simulink model "AttitudeControl_tune"  (R2017b)
settings: Solver=ode4  StartTime=0.0  StopTime=10  FixedStep=0.001  RelTol=1e-3
InitFcn:
  | Init_control
undefined symbols (not defined in the file): DiscIntNeverNeededParam, Kd_PITCH_AngleRate, Kd_ROLL_AngleRate, Kd_YAW_AngleRate, Ki_PITCH_AngleRate, Ki_ROLL_AngleRate, Ki_YAW_AngleRate, Kp_PITCH_ANGLE, Kp_PITCH_AngleRate, Kp_ROLL_ANGLE, Kp_ROLL_AngleRate, Kp_YAW_AngleRate, MAX_CONTROL_ANGLE_RATE_PITCH, MAX_CONTROL_ANGLE_RATE_ROLL, ModelInit_AngEuler, ModelInit_PosE, ModelInit_Rads, ModelInit_RateB, ModelInit_VelB, ModelParam_envGravityAcc, ModelParam_motorCr, ModelParam_motorJm, ModelParam_motorT, ModelParam_motorWb, ModelParam_rotorCm, ModelParam_rotorCt, ModelParam_uavCCm, ModelParam_uavCd, ModelParam_uavJ, ModelParam_uavMass, ModelParam_uavR, Saturation_I_RP_Max, Saturation_I_RP_Min, Saturation_I_Y_Max, Saturation_I_Y_Min
libraries: simulink x3, sharedutil x2
settings Model: Creator=wsh  LastModifiedBy=Mr Wang
settings OptimizationCC: MaxStackSize=64
settings DebuggingCC: ParameterTunabilityLossMsg=error
settings HardwareCC: ProdBitPerPointer=32  ProdBitPerSizeT=32  ProdBitPerPtrDiffT=32  ProdLargestAtomicInteger=Long  ProdLargestAtomicFloat=Double  ProdWordSize=32  ProdHWDeviceType=ARM Compatible->ARM Cortex
settings SFSimCC: MATLABDynamicMemAlloc=off
settings RTWCC: SystemTargetFile=ert.tlc  HardwareBoard=Pixhawk PX4  TemplateMakefile=ert_default_tmf  GenerateReport=on  Toolchain=Pixhawk Toolchain  IncludeHyperlinkInReport=on  LaunchReport=on  GenerateTraceInfo=on  GenerateTraceReport=on  GenerateTraceReportSl=on  GenerateTraceReportSf=on  GenerateTraceReportEml=on
settings CodeAppCC: ForceParamTrailComments=on  IgnoreCustomStorageClasses=off  OperatorAnnotations=on  SimulinkDataObjDesc=on  SFDataObjDesc=on  MATLABFcnDesc=on  InsertBlockDesc=on  StateflowObjectComments=on  MATLABSourceComments=on
settings ERTTargetCC: MultiwordLength=2048  ERTCustomFileTemplate=PX4_codertarget_file_process.tlc

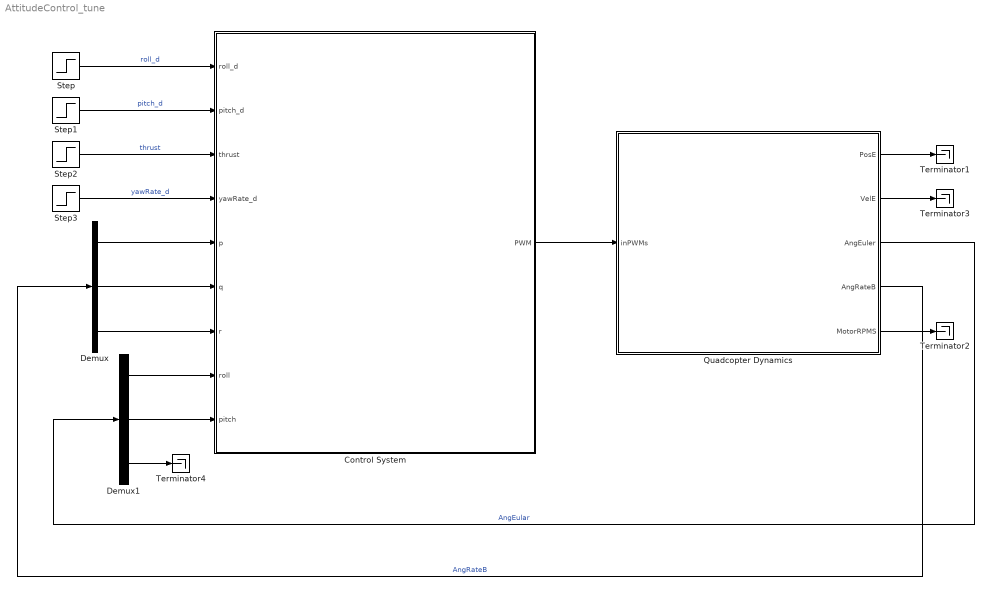
== system AttitudeControl_tune ==
  Control System : Subsystem
      mask Display: image('icon\pixhawk.png');
  Demux : Demux  Outputs=3
  Demux1 : Demux  Outputs=3
  Quadcopter Dynamics : Subsystem
      mask Display: image('./icon/F450.png');
  Step : Step  Time=0  After=0  SampleTime=0
  Step1 : Step  Time=0  After=0  SampleTime=0
  Step2 : Step  Time=0  After=0.6085  SampleTime=0
  Step3 : Step  Time=0  After=0  SampleTime=0
  Terminator{1..4} (4 alike) : Terminator
  wires:
  Quadcopter Dynamics/3(AngEuler) -> Demux1/1  "AngEular"
  Quadcopter Dynamics/4(AngRateB) -> Demux/1  "AngRateB"
  Demux/1 -> Control System/5(p)
  Demux/2 -> Control System/6(q)
  Demux/3 -> Control System/7(r)
  Demux1/1 -> Control System/8(roll)
  Demux1/3 -> Terminator4/1
  Demux1/2 -> Control System/9(pitch)
  Quadcopter Dynamics/1(PosE) -> Terminator1/1
  Quadcopter Dynamics/2(VelE) -> Terminator3/1
  Step1/1 -> Control System/2(pitch_d)  "pitch_d"
  Step/1 -> Control System/1(roll_d)  "roll_d"
  Step3/1 -> Control System/4(yawRate_d)  "yawRate_d"
  Step2/1 -> Control System/3(thrust)  "thrust"
  Quadcopter Dynamics/5(MotorRPMS) -> Terminator2/1
  Control System/1(PWM) -> Quadcopter Dynamics/1(inPWMs)

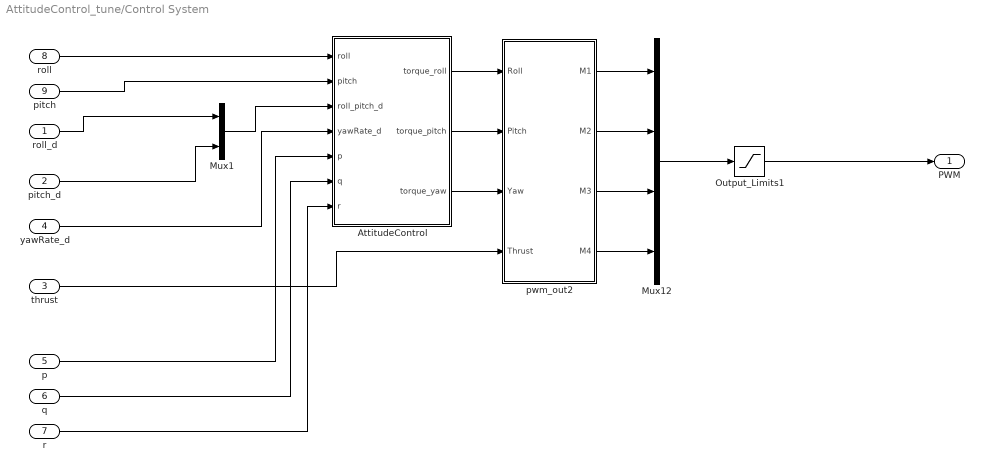
== system AttitudeControl_tune/Control System ==
  roll_d : Inport  PortDimensions=1
  pitch_d : Inport  Port=2  PortDimensions=1
  thrust : Inport  Port=3  PortDimensions=1
  yawRate_d : Inport  Port=4  PortDimensions=1
  p : Inport  Port=5  PortDimensions=1
  q : Inport  Port=6  PortDimensions=1
  r : Inport  Port=7  PortDimensions=1
  roll : Inport  Port=8  PortDimensions=1
  pitch : Inport  Port=9  PortDimensions=1
  AttitudeControl : Subsystem
  Mux1 : Mux  Inputs=2
  Mux12 : Mux
  Output_Limits1 : Saturate  UpperLimit=2000  LowerLimit=1000  LinearizeAsGain=off
  pwm_out2 : MATLAB Function  SystemSampleTime=0.004
  PWM : Outport
  wires:
  thrust/1 -> pwm_out2/4(Thrust)
  Mux12/1 -> Output_Limits1/1
  AttitudeControl/2(torque_pitch) -> pwm_out2/2(Pitch)
  AttitudeControl/1(torque_roll) -> pwm_out2/1(Roll)
  pwm_out2/1(M1) -> Mux12/1
  pwm_out2/3(M3) -> Mux12/3
  pwm_out2/2(M2) -> Mux12/2
  r/1 -> AttitudeControl/7(r)
  AttitudeControl/3(torque_yaw) -> pwm_out2/3(Yaw)
  Mux1/1 -> AttitudeControl/3(roll_pitch_d)
  q/1 -> AttitudeControl/6(q)
  yawRate_d/1 -> AttitudeControl/4(yawRate_d)
  p/1 -> AttitudeControl/5(p)
  pwm_out2/4(M4) -> Mux12/4
  pitch/1 -> AttitudeControl/2(pitch)
  roll/1 -> AttitudeControl/1(roll)
  Output_Limits1/1 -> PWM/1
  roll_d/1 -> Mux1/1
  pitch_d/1 -> Mux1/2

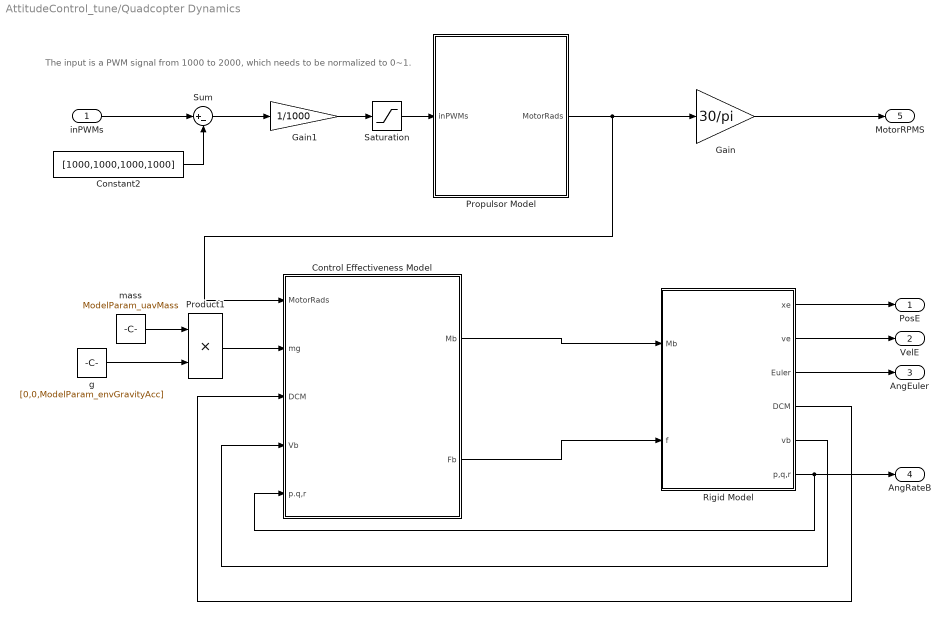
== system AttitudeControl_tune/Quadcopter Dynamics ==
  note: The input is a PWM signal from 1000 to 2000,
      | which needs to be normalized to 0~1.
  inPWMs : Inport
  Constant2 : Constant  Value=[1000,1000,1000,1000]
  Control Effectiveness Model : Subsystem
  Gain : Gain  Gain=30/pi
  Gain1 : Gain  Gain=1/1000
  Product1 : Product
  Propulsor Model : Subsystem
  Rigid Model : Subsystem
  Saturation : Saturate  UpperLimit=1  LowerLimit=0
  Sum : Sum  Inputs=|+-
  g : Constant  Value=[0,0,ModelParam_envGravityAcc]
  mass : Constant  Value=ModelParam_uavMass
  PosE : Outport
  VelE : Outport  Port=2
  AngEuler : Outport  Port=3
  AngRateB : Outport  Port=4
  MotorRPMS : Outport  Port=5
  wires:
  Saturation/1 -> Propulsor Model/1(inPWMs)
  Rigid Model/6("p,q,r ") -> Control Effectiveness Model/5(p.q,r), AngRateB/1
  mass/1 -> Product1/1
  Rigid Model/4(DCM) -> Control Effectiveness Model/3(DCM)
  Propulsor Model/1(MotorRads) -> Gain/1, Control Effectiveness Model/1(MotorRads)
  Gain1/1 -> Saturation/1
  Rigid Model/2(ve) -> VelE/1
  Sum/1 -> Gain1/1
  Product1/1 -> Control Effectiveness Model/2(mg)
  Rigid Model/5("vb ") -> Control Effectiveness Model/4(Vb)
  Rigid Model/1("xe ") -> PosE/1
  Rigid Model/3(Euler) -> AngEuler/1
  Control Effectiveness Model/1(Mb) -> Rigid Model/1(Mb)
  inPWMs/1 -> Sum/1
  Control Effectiveness Model/2(Fb) -> Rigid Model/2(f)
  Constant2/1 -> Sum/2
  g/1 -> Product1/2
  Gain/1 -> MotorRPMS/1

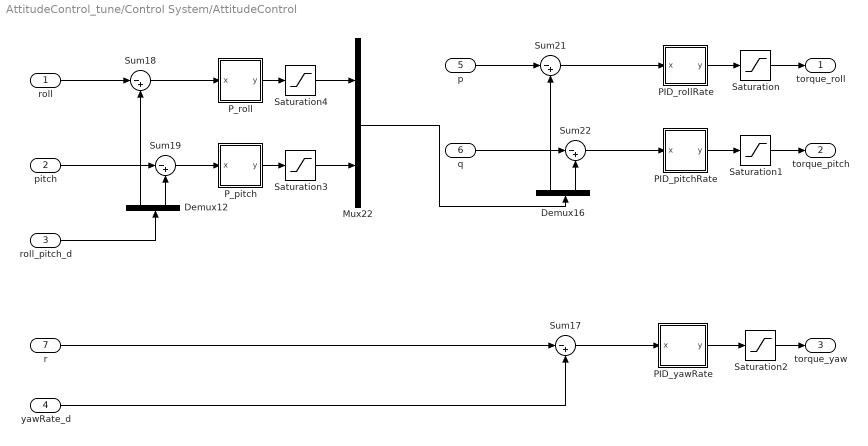
== system AttitudeControl_tune/Control System/AttitudeControl ==
  roll : Inport
  pitch : Inport  Port=2
  roll_pitch_d : Inport  Port=3
  yawRate_d : Inport  Port=4
  p : Inport  Port=5
  q : Inport  Port=6
  r : Inport  Port=7
  Demux12 : Demux  Outputs=2
  Demux16 : Demux  Outputs=2
  Mux22 : Mux  Inputs=2
  PID_pitchRate : Subsystem
  PID_rollRate : Subsystem
  PID_yawRate : Subsystem
  "P_pitch " : Subsystem
  "P_roll " : Subsystem
  Saturation : Saturate  UpperLimit=1  LowerLimit=-1
  Saturation1 : Saturate  UpperLimit=1  LowerLimit=-1
  Saturation2 : Saturate
  Saturation3 : Saturate  UpperLimit=MAX_CONTROL_ANGLE_RATE_PITCH  LowerLimit=-MAX_CONTROL_ANGLE_RATE_PITCH
  Saturation4 : Saturate  UpperLimit=MAX_CONTROL_ANGLE_RATE_ROLL  LowerLimit=-MAX_CONTROL_ANGLE_RATE_ROLL
  Sum{17..19,21..22} (5 alike) : Sum  Inputs=|-+
  torque_roll : Outport
  torque_pitch : Outport  Port=2
  torque_yaw : Outport  Port=3
  wires:
  r/1 -> Sum17/1
  Sum19/1 -> "P_pitch "/1(x)
  "P_pitch "/1(y) -> Saturation3/1
  "P_roll "/1(y) -> Saturation4/1
  roll/1 -> Sum18/1
  pitch/1 -> Sum19/1
  Sum18/1 -> "P_roll "/1(x)
  Sum22/1 -> PID_pitchRate/1(x)
  Sum17/1 -> PID_yawRate/1(x)
  p/1 -> Sum21/1
  q/1 -> Sum22/1
  Sum21/1 -> PID_rollRate/1(x)
  PID_pitchRate/1(y) -> Saturation1/1
  PID_rollRate/1(y) -> Saturation/1
  PID_yawRate/1(y) -> Saturation2/1
  roll_pitch_d/1 -> Demux12/1
  Saturation1/1 -> torque_pitch/1
  yawRate_d/1 -> Sum17/2
  Mux22/1 -> Demux16/1
  Saturation4/1 -> Mux22/1
  Saturation3/1 -> Mux22/2
  Saturation/1 -> torque_roll/1
  Saturation2/1 -> torque_yaw/1
  Demux16/1 -> Sum21/2
  Demux12/2 -> Sum19/2
  Demux12/1 -> Sum18/2
  Demux16/2 -> Sum22/2

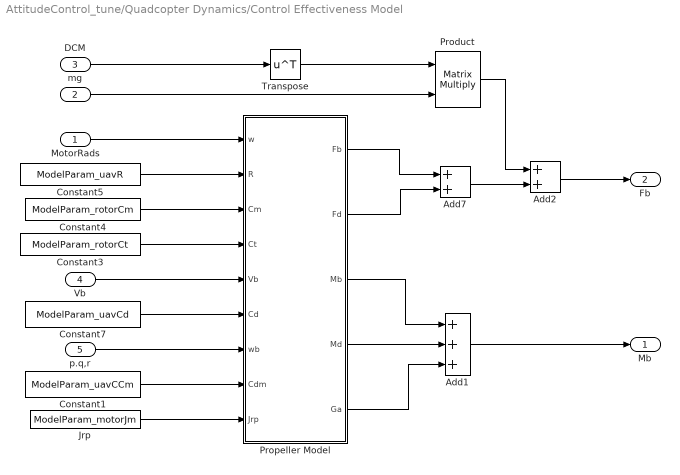
== system AttitudeControl_tune/Quadcopter Dynamics/Control Effectiveness Model ==
  MotorRads : Inport
  mg : Inport  Port=2
  DCM : Inport  Port=3
  Vb : Inport  Port=4
  p.q,r : Inport  Port=5
  Add1 : Sum  Inputs=+++
  Add2 : Sum
  Add7 : Sum
  Constant1 : Constant  Value=ModelParam_uavCCm
  Constant3 : Constant  Value=ModelParam_rotorCt
  Constant4 : Constant  Value=ModelParam_rotorCm
  Constant5 : Constant  Value=ModelParam_uavR
  Constant7 : Constant  Value=ModelParam_uavCd
  Jrp : Constant  Value=ModelParam_motorJm
  Product : Product  Multiplication=Matrix(*)
  Propeller Model : MATLAB Function  TreatAsAtomicUnit=on
  Transpose : Math  Operator=transpose  SaturateOnIntegerOverflow=on
  Mb : Outport
  Fb : Outport  Port=2
  wires:
  Add2/1 -> Fb/1
  Constant3/1 -> Propeller Model/4(Ct)
  Propeller Model/2(Fd) -> Add7/2
  Add7/1 -> Add2/2
  Propeller Model/1(Fb) -> Add7/1
  Product/1 -> Add2/1
  mg/1 -> Product/2
  DCM/1 -> Transpose/1
  Constant7/1 -> Propeller Model/6(Cd)
  Vb/1 -> Propeller Model/5(Vb)
  Constant5/1 -> Propeller Model/2(R)
  Constant4/1 -> Propeller Model/3(Cm)
  MotorRads/1 -> Propeller Model/1(w)
  Transpose/1 -> Product/1
  Propeller Model/3(Mb) -> Add1/1
  Propeller Model/4(Md) -> Add1/2
  Add1/1 -> Mb/1
  p.q,r/1 -> Propeller Model/7(wb)
  Constant1/1 -> Propeller Model/8(Cdm)
  Jrp/1 -> Propeller Model/9(Jrp)
  Propeller Model/5(Ga) -> Add1/3

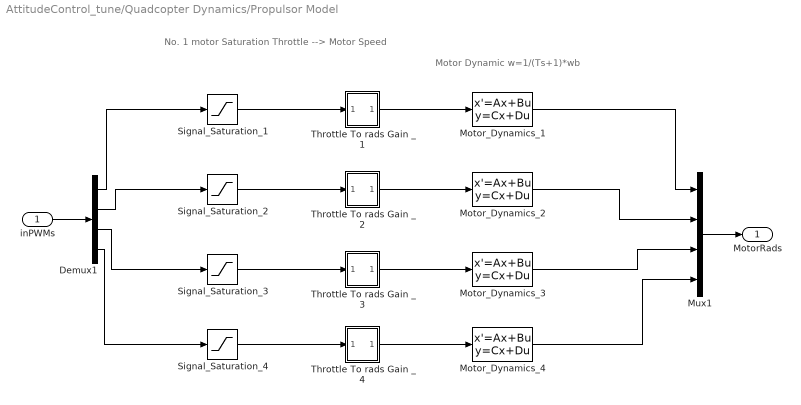
== system AttitudeControl_tune/Quadcopter Dynamics/Propulsor Model ==
  note: Motor Dynamic
      | w=1/(Ts+1)*wb
  note: No. 1 motor
      |
      |          Saturation             Throttle --> Motor Speed
  inPWMs : Inport
  Demux1 : Demux
  Motor_Dynamics_{1..4} (4 alike) : StateSpace  A=-1/ModelParam_motorT  C=1/ModelParam_motorT  D=0  InitialCondition=ModelInit_Rads*ModelParam_motorT
  Mux1 : Mux
  Signal_Saturation_{1..4} (4 alike) : Saturate  UpperLimit=1  LowerLimit=0
  Throttle To rads Gain _1 : Subsystem
  Throttle To rads Gain _2 : Subsystem
  Throttle To rads Gain _3 : Subsystem
  Throttle To rads Gain _4 : Subsystem
  MotorRads : Outport
  wires:
  Throttle To rads Gain _4/1(Out5) -> Motor_Dynamics_4/1
  Signal_Saturation_4/1 -> Throttle To rads Gain _4/1(In5)
  Signal_Saturation_3/1 -> Throttle To rads Gain _3/1(In5)
  Signal_Saturation_2/1 -> Throttle To rads Gain _2/1(In5)
  Motor_Dynamics_4/1 -> Mux1/4
  Motor_Dynamics_3/1 -> Mux1/3
  Motor_Dynamics_2/1 -> Mux1/2
  Motor_Dynamics_1/1 -> Mux1/1
  Signal_Saturation_1/1 -> Throttle To rads Gain _1/1(In5)
  Mux1/1 -> MotorRads/1
  Throttle To rads Gain _3/1(Out5) -> Motor_Dynamics_3/1
  Throttle To rads Gain _2/1(Out5) -> Motor_Dynamics_2/1
  Throttle To rads Gain _1/1(Out5) -> Motor_Dynamics_1/1
  inPWMs/1 -> Demux1/1
  Demux1/4 -> Signal_Saturation_4/1
  Demux1/3 -> Signal_Saturation_3/1
  Demux1/2 -> Signal_Saturation_2/1
  Demux1/1 -> Signal_Saturation_1/1

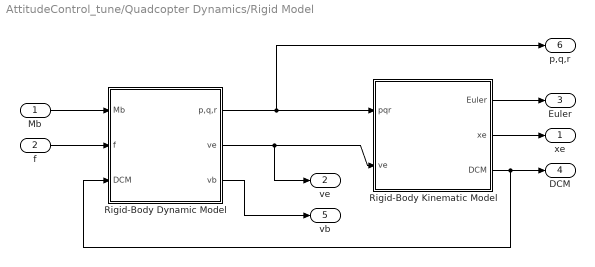
== system AttitudeControl_tune/Quadcopter Dynamics/Rigid Model ==
  Mb : Inport
  f : Inport  Port=2
  Rigid-Body Dynamic Model : Subsystem
  "Rigid-Body Kinematic Model " : Subsystem
  "xe " : Outport
  ve : Outport  Port=2
  Euler : Outport  Port=3
  DCM : Outport  Port=4
  "vb " : Outport  Port=5
  "p,q,r " : Outport  Port=6
  wires:
  Rigid-Body Dynamic Model/1("p,q,r ") -> "Rigid-Body Kinematic Model "/1(pqr), "p,q,r "/1
  "Rigid-Body Kinematic Model "/1(Euler) -> Euler/1
  "Rigid-Body Kinematic Model "/3(DCM) -> Rigid-Body Dynamic Model/3(DCM), DCM/1
  Mb/1 -> Rigid-Body Dynamic Model/1(Mb)
  f/1 -> Rigid-Body Dynamic Model/2(f)
  Rigid-Body Dynamic Model/2(ve) -> "Rigid-Body Kinematic Model "/2(ve), ve/1
  Rigid-Body Dynamic Model/3("vb ") -> "vb "/1
  "Rigid-Body Kinematic Model "/2("xe ") -> "xe "/1

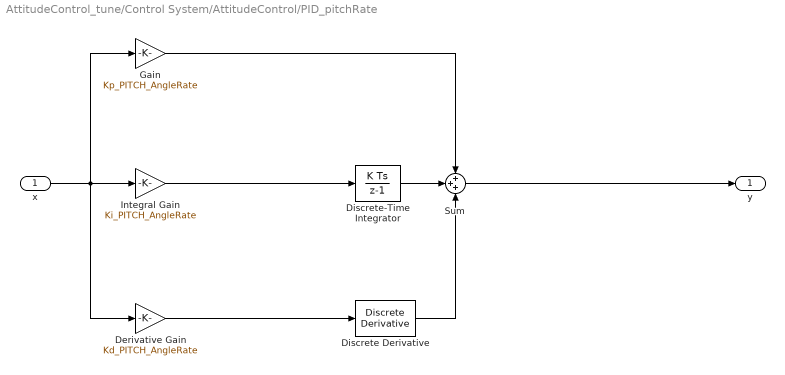
== system AttitudeControl_tune/Control System/AttitudeControl/PID_pitchRate ==
  x : Inport
  Derivative Gain : Gain  DisableCoverage=on  Gain=Kd_PITCH_AngleRate  ParamMin=-100  ParamMax=100  OutMin=-100  OutMax=100
  Discrete Derivative : simulink/Discrete/Discrete Derivative  gainval=1.0  ICPrevScaledInput=0.0  OutMin=[]  OutMax=[]  OutDataType=fixdt(1, 16)  OutScaling=2^-10  DoSatur=off
  Discrete-Time Integrator : DiscreteIntegrator  InitialConditionSetting=State (most efficient)  SampleTime=-1  LimitOutput=on  UpperSaturationLimit=Saturation_I_RP_Max  LowerSaturationLimit=Saturation_I_RP_Min  ICPrevOutput=DiscIntNeverNeededParam  ICPrevScaledInput=DiscIntNeverNeededParam
  Gain : Gain  Gain=Kp_PITCH_AngleRate
  Integral Gain : Gain  DisableCoverage=on  Gain=Ki_PITCH_AngleRate
  Sum : Sum  Inputs=+++
  y : Outport  InitialOutput=0
  wires:
  Discrete-Time Integrator/1 -> Sum/2
  Discrete Derivative/1 -> Sum/3
  Sum/1 -> y/1
  Gain/1 -> Sum/1
  Derivative Gain/1 -> Discrete Derivative/1
  Integral Gain/1 -> Discrete-Time Integrator/1
  x/1 -> Derivative Gain/1, Integral Gain/1, Gain/1

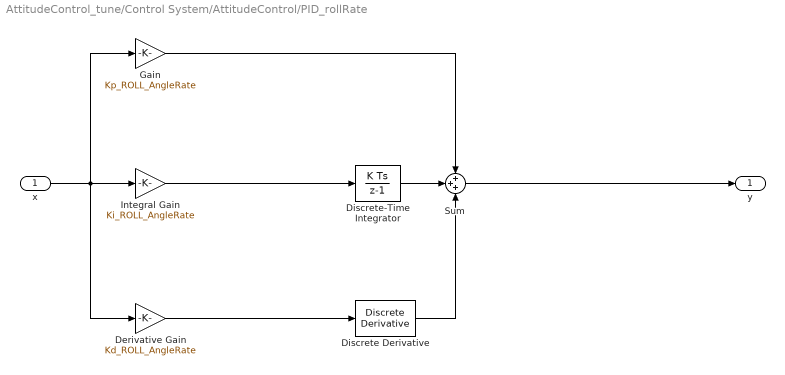
== system AttitudeControl_tune/Control System/AttitudeControl/PID_rollRate ==
  x : Inport
  Derivative Gain : Gain  DisableCoverage=on  Gain=Kd_ROLL_AngleRate  ParamMin=-100  ParamMax=100  OutMin=-100  OutMax=100
  Discrete Derivative : simulink/Discrete/Discrete Derivative  gainval=1.0  ICPrevScaledInput=0.0  OutMin=[]  OutMax=[]  OutDataType=fixdt(1, 16)  OutScaling=2^-10  DoSatur=off
  Discrete-Time Integrator : DiscreteIntegrator  InitialConditionSetting=State (most efficient)  SampleTime=-1  LimitOutput=on  UpperSaturationLimit=Saturation_I_RP_Max  LowerSaturationLimit=Saturation_I_RP_Min  ICPrevOutput=DiscIntNeverNeededParam  ICPrevScaledInput=DiscIntNeverNeededParam
  Gain : Gain  Gain=Kp_ROLL_AngleRate
  Integral Gain : Gain  DisableCoverage=on  Gain=Ki_ROLL_AngleRate
  Sum : Sum  Inputs=+++
  y : Outport  InitialOutput=0
  wires:
  x/1 -> Gain/1, Integral Gain/1, Derivative Gain/1
  Integral Gain/1 -> Discrete-Time Integrator/1
  Derivative Gain/1 -> Discrete Derivative/1
  Gain/1 -> Sum/1
  Sum/1 -> y/1
  Discrete Derivative/1 -> Sum/3
  Discrete-Time Integrator/1 -> Sum/2

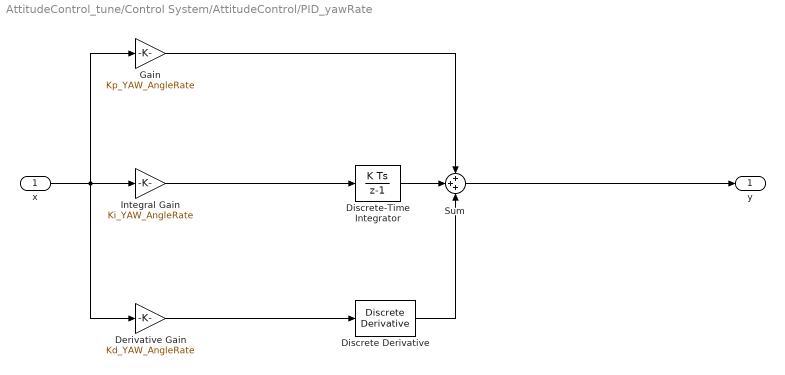
== system AttitudeControl_tune/Control System/AttitudeControl/PID_yawRate ==
  x : Inport
  Derivative Gain : Gain  DisableCoverage=on  Gain=Kd_YAW_AngleRate  ParamMin=-100  ParamMax=100  OutMin=-100  OutMax=100
  Discrete Derivative : simulink/Discrete/Discrete Derivative  gainval=1.0  ICPrevScaledInput=0.0  OutMin=[]  OutMax=[]  OutDataType=fixdt(1, 16)  OutScaling=2^-10  DoSatur=off
  Discrete-Time Integrator : DiscreteIntegrator  InitialConditionSetting=State (most efficient)  SampleTime=-1  LimitOutput=on  UpperSaturationLimit=Saturation_I_Y_Max  LowerSaturationLimit=Saturation_I_Y_Min  ICPrevOutput=DiscIntNeverNeededParam  ICPrevScaledInput=DiscIntNeverNeededParam
  Gain : Gain  Gain=Kp_YAW_AngleRate
  Integral Gain : Gain  DisableCoverage=on  Gain=Ki_YAW_AngleRate
  Sum : Sum  Inputs=+++
  y : Outport  InitialOutput=0
  wires:
  x/1 -> Gain/1, Integral Gain/1, Derivative Gain/1
  Integral Gain/1 -> Discrete-Time Integrator/1
  Derivative Gain/1 -> Discrete Derivative/1
  Gain/1 -> Sum/1
  Sum/1 -> y/1
  Discrete Derivative/1 -> Sum/3
  Discrete-Time Integrator/1 -> Sum/2

== system AttitudeControl_tune/Control System/AttitudeControl/P_pitch  ==
  x : Inport
  Gain : Gain  Gain=Kp_PITCH_ANGLE
  y : Outport  InitialOutput=0
  wires:
  x/1 -> Gain/1
  Gain/1 -> y/1

== system AttitudeControl_tune/Control System/AttitudeControl/P_roll  ==
  x : Inport
  Gain : Gain  Gain=Kp_ROLL_ANGLE
  y : Outport  InitialOutput=0
  wires:
  Gain/1 -> y/1
  x/1 -> Gain/1

== system AttitudeControl_tune/Quadcopter Dynamics/Propulsor Model/Throttle To rads Gain _1 ==
  In5 : Inport
  Constant : Constant  Value=ModelParam_motorWb
  Gain : Gain  Gain=ModelParam_motorCr
  Sum1 : Sum  Inputs=++|
  Out5 : Outport
  wires:
  Constant/1 -> Sum1/1
  Gain/1 -> Sum1/2
  In5/1 -> Gain/1
  Sum1/1 -> Out5/1

== system AttitudeControl_tune/Quadcopter Dynamics/Propulsor Model/Throttle To rads Gain _2 ==
  In5 : Inport
  Constant : Constant  Value=ModelParam_motorWb
  Gain : Gain  Gain=ModelParam_motorCr
  Sum1 : Sum  Inputs=++|
  Out5 : Outport
  wires:
  Sum1/1 -> Out5/1
  In5/1 -> Gain/1
  Gain/1 -> Sum1/2
  Constant/1 -> Sum1/1

== system AttitudeControl_tune/Quadcopter Dynamics/Propulsor Model/Throttle To rads Gain _3 ==
  In5 : Inport
  Constant : Constant  Value=ModelParam_motorWb
  Gain : Gain  Gain=ModelParam_motorCr
  Sum1 : Sum  Inputs=++|
  Out5 : Outport
  wires:
  Constant/1 -> Sum1/1
  Gain/1 -> Sum1/2
  In5/1 -> Gain/1
  Sum1/1 -> Out5/1

== system AttitudeControl_tune/Quadcopter Dynamics/Propulsor Model/Throttle To rads Gain _4 ==
  In5 : Inport
  Constant : Constant  Value=ModelParam_motorWb
  Gain : Gain  Gain=ModelParam_motorCr
  Sum1 : Sum  Inputs=++|
  Out5 : Outport
  wires:
  Sum1/1 -> Out5/1
  In5/1 -> Gain/1
  Gain/1 -> Sum1/2
  Constant/1 -> Sum1/1

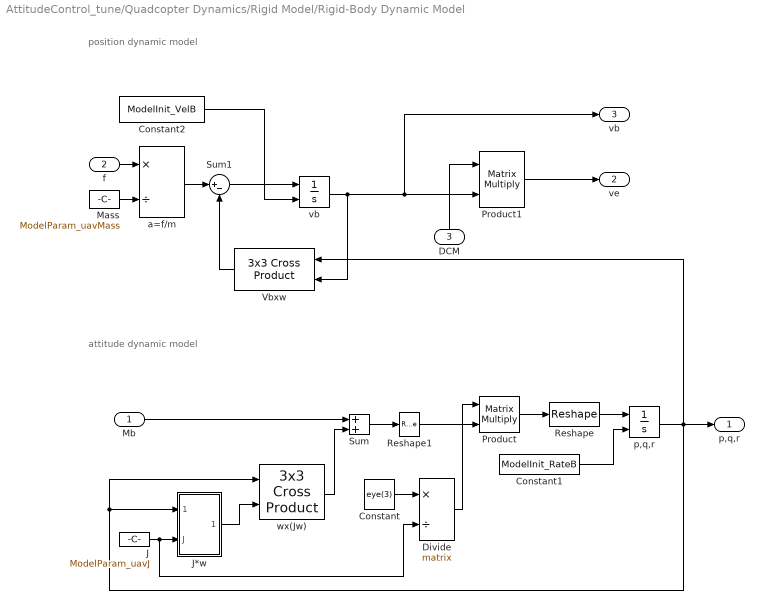
== system AttitudeControl_tune/Quadcopter Dynamics/Rigid Model/Rigid-Body Dynamic Model ==
  note: attitude dynamic model
  note: position dynamic model
  Mb : Inport
  f : Inport  Port=2
  DCM : Inport  Port=3
  " Mass " : Constant  Value=ModelParam_uavMass
  Constant : Constant  Value=eye(3)
  Constant1 : Constant  Value=ModelInit_RateB
  Constant2 : Constant  Value=ModelInit_VelB
  Divide : Product  Inputs=*/  Multiplication=Matrix(*)
  "J " : Constant  Value=ModelParam_uavJ
  J*w : Subsystem
  Product : Product  Multiplication=Matrix(*)
  Product1 : Product  Multiplication=Matrix(*)
  Reshape : Reshape  OutputDimensionality=Customize  OutputDimensions=[3,1]
  Reshape1 : Reshape  OutputDimensionality=Column vector (2-D)
  Sum : Sum  Inputs=2
  Sum1 : Sum  Inputs=|+-
  Vbxw : sharedutil/3x3 Cross Product
      settings: SourceProductBaseCode=AE
  a=f/m : Product  Inputs=*/
  p,q,r : Integrator  InitialConditionSource=external
  vb : Integrator  InitialConditionSource=external
  wx(Jw) : sharedutil/3x3 Cross Product
      settings: SourceProductBaseCode=AE
  "p,q,r " : Outport
  ve : Outport  Port=2
  "vb " : Outport  Port=3
  wires:
  Product/1 -> Reshape/1
  Reshape1/1 -> Product/2
  Constant/1 -> Divide/1
  Divide/1 -> Product/1
  Sum/1 -> Reshape1/1
  "J "/1 -> Divide/2, J*w/2(J)
  p,q,r/1 -> "p,q,r "/1, J*w/1(p q r), wx(Jw)/1, Vbxw/1
  J*w/1("J*w ") -> wx(Jw)/2
  Mb/1 -> Sum/1
  wx(Jw)/1 -> Sum/2
  Constant2/1 -> vb/2
  f/1 -> a=f/m/1
  Product1/1 -> ve/1
  Vbxw/1 -> Sum1/2
  a=f/m/1 -> Sum1/1
  Sum1/1 -> vb/1
  vb/1 -> Product1/2, "vb "/1, Vbxw/2
  " Mass "/1 -> a=f/m/2
  DCM/1 -> Product1/1
  Reshape/1 -> p,q,r/1
  Constant1/1 -> p,q,r/2

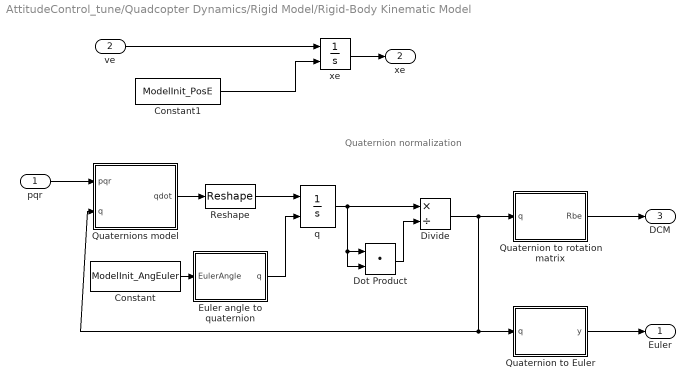
== system AttitudeControl_tune/Quadcopter Dynamics/Rigid Model/Rigid-Body Kinematic Model  ==
  note: Quaternion
      | normalization
  pqr : Inport
  ve : Inport  Port=2
  Constant : Constant  Value=ModelInit_AngEuler
  Constant1 : Constant  Value=ModelInit_PosE
  Divide : Product  Inputs=*/
  Dot Product : DotProduct  InputSameDT=on  OutDataTypeStr=Inherit: Inherit via internal rule
  Euler angle to quaternion : MATLAB Function
  Quaternion to Euler : MATLAB Function
  Quaternion to rotation matrix : MATLAB Function
  Quaternions model : MATLAB Function  TreatAsAtomicUnit=on
  Reshape : Reshape  OutputDimensionality=Customize  OutputDimensions=[4,1]
  q : Integrator  InitialConditionSource=external
  xe : Integrator  InitialConditionSource=external
  Euler : Outport
  "xe " : Outport  Port=2
  DCM : Outport  Port=3
  wires:
  Divide/1 -> Quaternion to rotation matrix/1(q), Quaternion to Euler/1(q), Quaternions model/2(q)
  Dot Product/1 -> Divide/2
  pqr/1 -> Quaternions model/1(pqr)
  q/1 -> Dot Product/1, Dot Product/2, Divide/1
  Quaternions model/1(qdot) -> Reshape/1
  Quaternion to rotation matrix/1(Rbe) -> DCM/1
  Quaternion to Euler/1(y) -> Euler/1
  Constant/1 -> Euler angle to quaternion/1(EulerAngle)
  Euler angle to quaternion/1(q) -> q/2
  Reshape/1 -> q/1
  ve/1 -> xe/1
  xe/1 -> "xe "/1
  Constant1/1 -> xe/2

== system AttitudeControl_tune/Quadcopter Dynamics/Rigid Model/Rigid-Body Dynamic Model/J*w ==
  p q r : Inport
  J : Inport  Port=2
  J*w : Product  Multiplication=Matrix(*)
  "J*w " : Outport
  wires:
  J*w/1 -> "J*w "/1
  J/1 -> J*w/1
  p q r/1 -> J*w/2

== matlab function AttitudeControl_tune/Quadcopter Dynamics/Rigid Model/Rigid-Body Kinematic Model /Quaternion to rotation matrix ==
  data: q input; Rbe output
function Rbe = fcn(q)
%Function description;
%  The rotation matrix of the body coordinate system to the geodetic coordinate system is obtained from the quaternion
Rbe = [q(1)*q(1) + q(2)*q(2) - q(3)*q(3) - q(4)*q(4), 2*(q(2)*q(3) - q(1)*q(4)), 2*(q(2)*q(4) + q(1)*q(3))
       2*(q(2)*q(3) + q(1)*q(4)), q(1)*q(1) - q(2)*q(2) + q(3)*q(3) - q(4)*q(4), 2*(q(3)*q(4) - q(1)*q(2))
       2*(q(2)*q(4) - q(1)*q(3)), 2*(q(3)*q(4) + q(1)*q(2)), q(1)*q(1) - q(2)*q(2) - q(3)*q(3) + q(4)*q(4)];

== matlab function AttitudeControl_tune/Quadcopter Dynamics/Rigid Model/Rigid-Body Kinematic Model /Quaternion to Euler ==
  data: q input; y output
function y = fcn(q)
 %Function description;
%  Quaternion to Euler
phi = atan2(2*(q(1)*q(2) + q(3)*q(4)), (1 - 2*(q(2)*q(2) + q(3)*q(3))));
theta = asin(2*(q(1)*q(3) - q(2)*q(4)));
psi = atan2(2*(q(1)*q(4) + q(2)*q(3)), (1 - 2*(q(3)*q(3) + q(4)*q(4))));
y = [phi theta psi];

== matlab function AttitudeControl_tune/Quadcopter Dynamics/Rigid Model/Rigid-Body Kinematic Model /Quaternions model ==
  data: pqr input; qdot output; q input
function qdot = fcn(pqr, q)
%Function description;
%  Quaternions model
qdot = 0.5*[0, -pqr(1), -pqr(2), -pqr(3); pqr(1), 0, pqr(3), -pqr(2); pqr(2), -pqr(3), 0, pqr(1); pqr(3), pqr(2), -pqr(1), 0]*q;

== matlab function AttitudeControl_tune/Quadcopter Dynamics/Rigid Model/Rigid-Body Kinematic Model /Euler angle to quaternion ==
  data: EulerAngle input; q output
function q = fcn(EulerAngle)
%Function description;
%  Get quaternion from Euler angle
q0 =  cos(EulerAngle(1)/2)*cos(EulerAngle(2)/2)*cos(EulerAngle(3)/2) + sin(EulerAngle(1)/2)*sin((EulerAngle(2)/2))*sin((EulerAngle(3)/2));
q1 = -sin(EulerAngle(1)/2)*cos(EulerAngle(2)/2)*cos(EulerAngle(3)/2) + cos(EulerAngle(1)/2)*sin((EulerAngle(2)/2))*sin((EulerAngle(3)/2));
q2 = -cos(EulerAngle(1)/2)*sin(EulerAngle(2)/2)*cos(EulerAngle(3)/2) - sin(EulerAngle(1)/2)*cos((EulerAngle(2)/2))*sin((EulerAngle(3)/2));
q3 = -cos(EulerAngle(1)/2)*cos(EulerAngle(2)/2)*sin(EulerAngle(3)/2) + sin(EulerAngle(1)/2)*sin((EulerAngle(2)/2))*cos((EulerAngle(3)/2));
q = [q0 q1 q2 q3]';

== matlab function AttitudeControl_tune/Quadcopter Dynamics/Control Effectiveness Model/Propeller Model ==
  data: w input; R input; Fb output; Fd output; Mb output; Cm input; Ct input; Vb input; Cd input; wb input; Md output; Cdm input; Jrp input; Ga output
function [Fb, Fd, Mb, Md, Ga] = fcn(w, R, Cm, Ct, Vb, Cd,wb, Cdm, Jrp)
 %Function description;
 %  According to the rotational speed, the force and torque provided by the propeller 
 %  to the quadrotor-X aircraft are calculated. The distribution of the quadrotor motor is as follows:
 %3↓   1↑
 %  \ /
 %  / \
 %2↑   4↓
 %↑ stands for counterclockwise and ↓stands for clockwise
 %Input：
 %  w: Motor speed，unit：rad/s
 %  R: Body radius(m)
 %  Cm: torque coefficient
 %  Ct: thrust coefficient
 %  Vb: Aircraft speed in the body coordinate system
 %  Cd: Damping coefficient
 %  wb: Angular velocity in the body coordinate system
 %  Cdm: Damping moment coefficient vector
 %  Jrp:  Moment of inertia of motor rotor + propeller
 %Output:
 %  Fb: thrust under the body coordinate system
 %  Fd: air resistance under the body coordinate system
 %  Mb: torque under the body coordinate system
 %  Md: aerodynamic moment
 %  Ga: gyro moment
 M_rctcm = [-sin(pi/4)*R*Ct, sin(pi/4)*R*Ct, sin(pi/4)*R*Ct, -sin(pi/4)*R*Ct;
            sin(pi/4)*R*Ct, -sin(pi/4)*R*Ct, sin(pi/4)*R*Ct, -sin(pi/4)*R*Ct;
            Cm, Cm, -Cm, -Cm];
 Mb = M_rctcm*(w.^2);  %torque
 
 Fb = [0; 0; -sum(Ct*(w.^2))];  %thrust
 Fd = -Cd*Vb.*abs(Vb)*0.5;  %aerodynamic force
 Md = -Cdm.*wb.*abs(wb);  %aerodynamic moment
 %Calculating gyro moment
 Ga = zeros(3,1);
 Ga(1) = Jrp*wb(2)*( w(1) + w(2) - w(3) - w(4));
 Ga(2) = Jrp*wb(1)*(-w(1) - w(2) + w(3) + w(4));
end

== matlab function AttitudeControl_tune/Control System/pwm_out2 ==
  data: Roll input; M1 output; Pitch input; Yaw input; Thrust input; M2 output; M3 output; M4 output
function [M1, M2, M3, M4] = motor_mixer(Roll, Pitch, Yaw, Thrust)
%Function description;
%  Assign the attitude controller output to the motor control. The multi-rotor type is quadrotor-X type,
%  and the propeller serial number is as follows:
%3↓   1↑
%  \ /
%  / \
%2↑   4↓
%↑ stands for counterclockwise and ↓stands for clockwise
%Input：
%  Roll, Pitch, Yaw: Attitude controller outputs.
%  Thrust

idle_PWM = 1000;
scale = 1000;
%the output PWMs range from 1000 to 2000
M1 = (Thrust - Roll + Pitch + Yaw) * scale + idle_PWM;
M2 = (Thrust + Roll - Pitch + Yaw) * scale + idle_PWM;
M3 = (Thrust + Roll + Pitch - Yaw) * scale + idle_PWM;
M4 = (Thrust - Roll - Pitch - Yaw) * scale + idle_PWM;
